simulink model "Modellierung_elekt_mech"  (R2017b)
settings: Solver=ode45  StartTime=0.0  StopTime=10  FixedStep=0.0001  MaxStep=1e-4  RelTol=1e-3  EnableMultiTasking=on
values from neighbouring files (symbols this model uses):
  C = 1e-3    (= 0.001)    [Modellierung_Konstanten.m]
  CF = 1e4    (= 10000)    [Modellierung_Konstanten.m]
  CR = 1e2    (= 100)    [Modellierung_Konstanten.m]
  L1 = 1e-3    (= 0.001)    [Modellierung_Konstanten.m]
  L2 = 1e-3    (= 0.001)    [Modellierung_Konstanten.m]
  m1 = 1e3    (= 1000)    [Modellierung_Konstanten.m]
  m2 = 2e2    (= 200)    [Modellierung_Konstanten.m]
  R = 50    [Modellierung_Konstanten.m]
undefined symbols (not defined in the file or in its folder): sigbuilder_block
settings Model: Creator=jbaur  LastModifiedBy=jbaur
settings DataIOCC: ExternalInput=X1  SaveFormat=StructureWithTime  SignalLoggingName=sigsOut
settings OptimizationCC: DefaultParameterBehavior=Inlined  InlineInvariantSignals=on  BufferReuse=off  ExpressionDepthLimit=2147483647  InitFltsAndDblsToZero=on  LifeSpan=inf
settings DebuggingCC: SaveWithParameterizedLinksMsg=none  SignalResolutionControl=TryResolveAllWithWarning  MultiTaskDSMMsg=warning  MultiTaskCondExecSysMsg=none  StateNameClashWarn=warning  InitInArrayFormatMsg=none  SFUnexpectedBacktrackingDiag=warning  SFNoUnconditionalDefaultTransitionDiag=warning  SFExecutionAtInitializationDiag=none
settings HardwareCC: ProdBitPerInt=16  ProdBitPerPointer=16  ProdBitPerSizeT=16  ProdBitPerPtrDiffT=16  ProdEndianess=Unspecified  ProdWordSize=8  ProdShiftRightIntArith=off  ProdHWDeviceType=Intel->8051 Compatible
settings ModelReferenceCC: PropagateSignalLabelsOutOfModel=off
settings CodeAppCC: StateflowObjectComments=on
settings GRTTargetCC: TargetFcnLib=ansi_tfl_tmw.mat  TargetLangStandard=C89/C90 (ANSI)  ModelReferenceCompliant=off  GeneratePreprocessorConditionals=Disable all  CombineOutputUpdateFcns=off  MatFileLogging=off  GRTInterface=on
settings ConfigComp: CovMetricSettings=dw  CovHtmlReporting=on  CovSaveCumulativeToWorkspaceVar=on  CovSaveSingleToWorkspaceVar=on  CovExternalEMLEnable=off  CovSFcnEnable=off

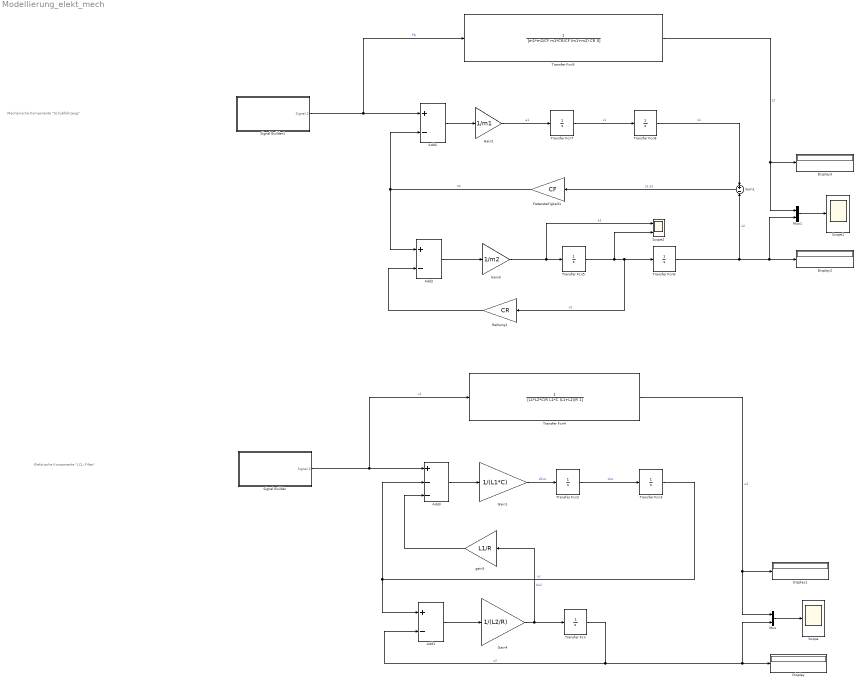
== system Modellierung_elekt_mech ==
  note: Elektrische Komponente "LCL-Filter"
  note: Mechanische Komponente "Schubfahrzeug"
  Add1 : Sum  Inputs=+-
  Add2 : Sum  Inputs=+-
  Add3 : Sum  Inputs=+--
  Add4 : Sum  Inputs=+-
  Display{,1..3} (4 alike) : Display
  Federsteifigkeit1 : Gain  Gain=CF
  Gain1 : Gain  Gain=1/(L1*C)
  Gain2 : Gain  Gain=1/m1
  Gain3 : Gain  Gain=1/m2
  Gain4 : Gain  Gain=1/(L2/R)
  Mux : Mux  Inputs=2
  Mux1 : Mux  Inputs=2
  Reibung1 : Gain  Gain=CR
  Scope : Scope
  Scope1 : Scope
  Scope2 : Scope  NumInputPorts=2
  Signal Builder : Subsystem  Tag=STV Subsys  LoadFcn=sigbuilder_block('load');  StartFcn=sigbuilder_block('start');  StopFcn=sigbuilder_block('stop');  ClipboardFcn=sigbuilder_block('clipboard');  mask(Sigbuilder block){tuvar=[0:10]}
      mask help: Simulink:masks:SigbuilderBlock_MD
      mask init:
      | if ~strcmp(get_param(bdroot(gcbh),'SimulationStatus'),'stopped') tuvar = sigbuilder_block('maskInit'); end
      settings: CopyFcn=sigbuilder_block('copy');  DeleteFcn=sigbuilder_block('delete');  ModelCloseFcn=sigbuilder_block('modelClose');  PreSaveFcn=sigbuilder_block('preSave');  PauseFcn=sigbuilder_block('pause');  ContinueFcn=sigbuilder_block('continue');  NameChangeFcn=sigbuilder_block('namechange');  OpenFcn=sigbuilder_block('open',[437.6 199.2 550.4 400 ]);  CloseFcn=sigbuilder_block('close');
      mask Display: plot(0, 0, 100, 100,[2, 2, 32, 32, 2], [68, 8, 8, 68, 68],[32, 2], [38, 38], [32, 19, 2],[53, 60, 44], [32, 17, 17, 2],[16, 16, 31, 31]);txt = getActiveGroup(gcbh);text(2, 100, txt,'verticalAlignment', 'top');
  Signal Builder1 : Subsystem  Tag=STV Subsys  LoadFcn=sigbuilder_block('load');  StartFcn=sigbuilder_block('start');  StopFcn=sigbuilder_block('stop');  ClipboardFcn=sigbuilder_block('clipboard');  mask(Sigbuilder block){tuvar=[0:10]}
      mask help: Simulink:masks:SigbuilderBlock_MD
      mask init:
      | if ~strcmp(get_param(bdroot(gcbh),'SimulationStatus'),'stopped') tuvar = sigbuilder_block('maskInit'); end
      settings: CopyFcn=sigbuilder_block('copy');  DeleteFcn=sigbuilder_block('delete');  ModelCloseFcn=sigbuilder_block('modelClose');  PreSaveFcn=sigbuilder_block('preSave');  PauseFcn=sigbuilder_block('pause');  ContinueFcn=sigbuilder_block('continue');  NameChangeFcn=sigbuilder_block('namechange');  OpenFcn=sigbuilder_block('open',[437.6 199.2 550.4 400 ]);  CloseFcn=sigbuilder_block('close');
      mask Display: plot(0, 0, 100, 100,[2, 2, 32, 32, 2], [68, 8, 8, 68, 68],[32, 2], [38, 38], [32, 19, 2],[53, 60, 44], [32, 17, 17, 2],[16, 16, 31, 31]);txt = getActiveGroup(gcbh);text(2, 100, txt,'verticalAlignment', 'top');
  Sum1 : Sum  Inputs=+|-
  Transfer Fcn{,2..3,5..8} (7 alike) : TransferFcn  Denominator=[1 0]
  Transfer Fcn4 : TransferFcn  Denominator=[L1*L2*C/R L1*C (L1+L2)/R 1]
  Transfer Fcn9 : TransferFcn  Denominator=[m1*m2/CF m1*CR/CF (m1+m2) CR 0]
  gain5 : Gain  Gain=L1/R
  wires:
  Gain4/1 -> gain5/1, Transfer Fcn/1  "du2"
  Add1/1 -> Gain4/1
  Transfer Fcn/1 -> Add1/2, Display/1, Mux/2  "u2"
  Gain1/1 -> Transfer Fcn2/1  "d2uc"
  Add3/1 -> Gain1/1
  Signal Builder/1(Signal 2) -> Transfer Fcn4/1, Add3/1  "u1"
  Transfer Fcn2/1 -> Transfer Fcn3/1  "duc"
  Transfer Fcn3/1 -> Add1/1, Add3/2  "uc"
  Mux/1 -> Scope/1
  Transfer Fcn5/1 -> Scope2/2, Reibung1/1, Transfer Fcn6/1  "v2"
  Transfer Fcn6/1 -> Sum1/2, Display2/1, Mux1/2  "s2"
  Gain3/1 -> Scope2/1, Transfer Fcn5/1  "a1"
  Add2/1 -> Gain3/1
  Reibung1/1 -> Add2/2
  Gain2/1 -> Transfer Fcn7/1  "a1"
  Add4/1 -> Gain2/1
  Federsteifigkeit1/1 -> Add2/1, Add4/2  "FF"
  Signal Builder1/1(Signal 2) -> Transfer Fcn9/1, Add4/1  "FA"
  Transfer Fcn7/1 -> Transfer Fcn8/1  "v1"
  Transfer Fcn8/1 -> Sum1/1  "s1"
  Sum1/1 -> Federsteifigkeit1/1  "s1-s2"
  Mux1/1 -> Scope1/1
  Transfer Fcn9/1 -> Display3/1, Mux1/1  "s2"
  gain5/1 -> Add3/3
  Transfer Fcn4/1 -> Mux/1, Display1/1  "u2"

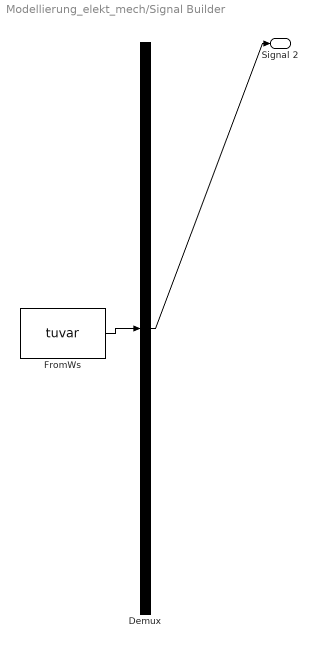
== system Modellierung_elekt_mech/Signal Builder ==
  Demux : Demux  Tag=STV Demux  Outputs=1
  FromWs : FromWorkspace  Tag=STV FromWs  VariableName=tuvar  SampleTime=0
      SigBuilderData=|
      | common.afterFinalStr = 'Extrapolate'
      | common.sampleTime = 0
      | dataSet.timeRange = [0 10]
      | dataSet.name = 'Group 1'
      | sbobj.Groups.Name = 'Group 1'
      | sbobj.Groups.Signals.Name = 'Signal 2'
      | sbobj.Groups.Signals.XData = [0 1 1 10]
      | sbobj.Groups.Signals.YData = [0 0 5 5]
  Signal 2 : Outport  Tag=STV Outport
  wires:
  FromWs/1 -> Demux/1
  Demux/1 -> Signal 2/1

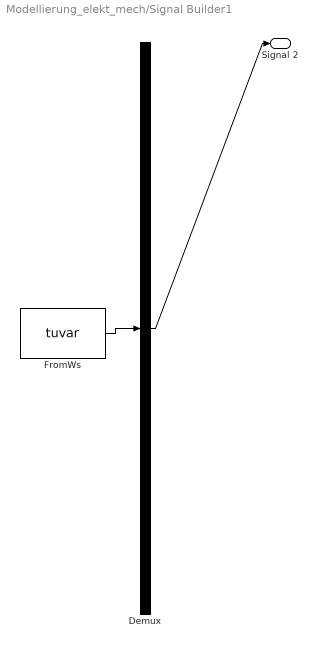
== system Modellierung_elekt_mech/Signal Builder1 ==
  Demux : Demux  Tag=STV Demux  Outputs=1
  FromWs : FromWorkspace  Tag=STV FromWs  VariableName=tuvar  SampleTime=0
      SigBuilderData=|
      | common.afterFinalStr = 'Extrapolate'
      | common.sampleTime = 0
      | dataSet.timeRange = [0 10]
      | dataSet.name = 'Group 1'
      | sbobj.Groups.Name = 'Group 1'
      | sbobj.Groups.Signals.Name = 'Signal 2'
      | sbobj.Groups.Signals.XData = [0 1 1 5 5 10]
      | sbobj.Groups.Signals.YData = [0 0 500 500 0 0]
  Signal 2 : Outport  Tag=STV Outport
  wires:
  FromWs/1 -> Demux/1
  Demux/1 -> Signal 2/1
